simulink model "lab1s"  (R2024b)
settings: Solver=VariableStepAuto  StartTime=0.0  StopTime=10.0  RelTol=1e-3
values from neighbouring files (symbols this model uses):
  Cvp = cpp * roo * Vp    (= 75000)    [lab1.m]
  Cvw = cpp * roo * Vw    (= 300000)    [lab1.m]
  czas_skok = 1500    [lab1.m]
  dPg = 1/10 * PgN    (= 1000)    [lab1.m]
  dTzew = 0    [lab1.m]
  K1 = a * Kp    (= 240)    [lab1.m]
  Kd = (Kp * (TwewN - TpN)) / (TpN - TzewN)    (= 11.4285714286)    [lab1.m]
  Kp = PgN / (a * (TwewN - TzewN) + (TwewN - TpN))    (= 80)    [lab1.m]
  Pg0 = tabl_Pg(i)    [lab1.m]
  Tp0 = (Kp / (Kp + Kd)) * (Pg0 / (K1 + (Kp * Kd) / (Kp + Kd))) + Tzew0    (= 15)    [lab1.m]
  Twew0 = (Pg0 / (K1 + (Kp * Kd) / (Kp + Kd))) + Tzew0    (= 20)    [lab1.m]
  Tzew0 = tab_Tzew(i)    [lab1.m]
settings Model: Creator=Adam  LastModifiedBy=Adam

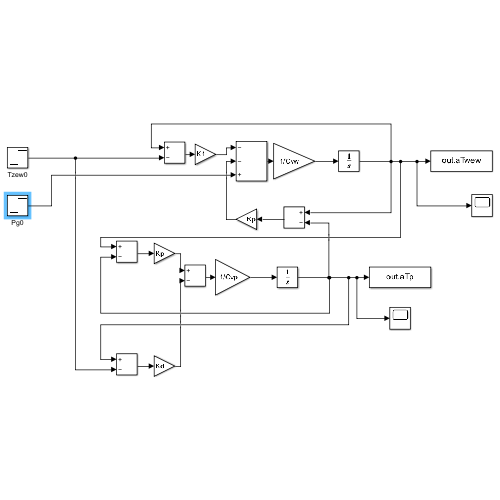
[thumbnail: Simulink's stored preview of the top-level diagram]
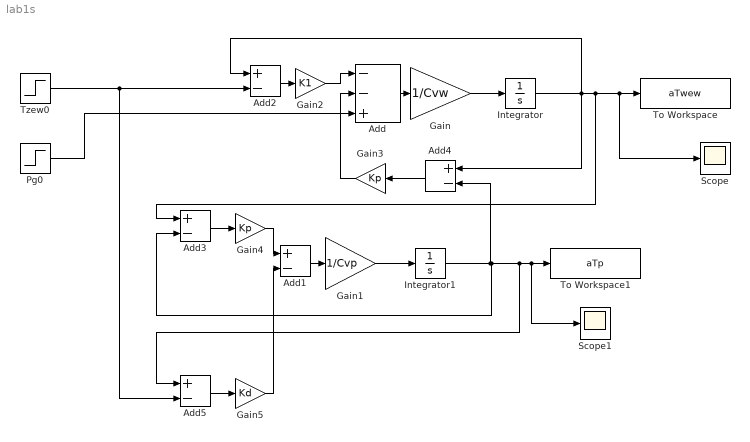
== system lab1s ==
  Add : Sum  Inputs=--+
  Add{1..5} (5 alike) : Sum  Inputs=+-
  Gain : Gain  Gain=1/Cvw
  Gain1 : Gain  Gain=1/Cvp
  Gain2 : Gain  Gain=K1
  Gain3 : Gain  Gain=Kp
  Gain4 : Gain  Gain=Kp
  Gain5 : Gain  Gain=Kd
  Integrator : Integrator  InitialCondition=Twew0
  Integrator1 : Integrator  InitialCondition=Tp0
  Pg0 : Step  Time=czas_skok  Before=Pg0  After=Pg0 + dPg  SampleTime=0
  Scope : Scope
  Scope1 : Scope
  To Workspace : ToWorkspace  VariableName=aTwew  SampleTime=-1
  To Workspace1 : ToWorkspace  VariableName=aTp  SampleTime=-1
  Tzew0 : Step  Time=czas_skok  Before=Tzew0  After=Tzew0 + dTzew  SampleTime=0
  wires:
  Add/1 -> Gain/1
  Gain/1 -> Integrator/1
  Add1/1 -> Gain1/1
  Gain1/1 -> Integrator1/1
  Integrator/1 -> Add4/1, Add2/1, Add3/1, Scope/1, To Workspace/1
  Integrator1/1 -> Add4/2, Add3/2, Add5/1, Scope1/1, To Workspace1/1
  Tzew0/1 -> Add5/2, Add2/2
  Add2/1 -> Gain2/1
  Gain2/1 -> Add/1
  Gain3/1 -> Add/2
  Add3/1 -> Gain4/1
  Gain4/1 -> Add1/1
  Add5/1 -> Gain5/1
  Gain5/1 -> Add1/2
  Add4/1 -> Gain3/1
  Pg0/1 -> Add/3
